simulink model "Qbot_2022a"  (R2023a)
settings: Solver=ode1  StartTime=0.0  StopTime=inf  FixedStep=1/60  RelTol=1e-3
PostLoadFcn:
  | qlabs_setup
model workspace: external: MATLAB File Qbot_2022a_saveas.m (data not in the file)
values from neighbouring files (symbols this model uses):
  D = 0.393    [param.m]
  kd1 = 1    [param.m]
  kd2 = kd1    (= 1)    [param.m]
  kp1 = 2    [param.m]
  kp2 = kp1    (= 2)    [param.m]
  R = 0.04445    [param.m]
  Tinv = inv(T)    [param.m]
  v0 = sqrt(xdr0.^2+ydr0.^2)    [param.m]
  wlmax = wrmax    (= 8)    [param.m]
  wrmax = 8.0    (= 8)    [param.m]
  X0 = [0 0 0]'    [param.m]
libraries: quarc_library x11, dspsigops x1
settings Model: SimulationMode=external  ExtModeTrigDuration=10000  Creator=mbohra  LastModifiedBy=surya
settings DebuggingCC: UnderspecifiedInitializationDetection=Classic  MergeDetectMultiDrivingBlocksExec=none
settings ModelReferenceCC: PropagateSignalLabelsOutOfModel=off

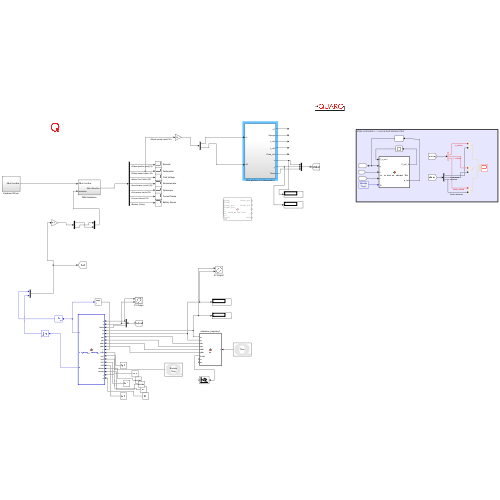
[thumbnail: Simulink's stored preview of the top-level diagram]
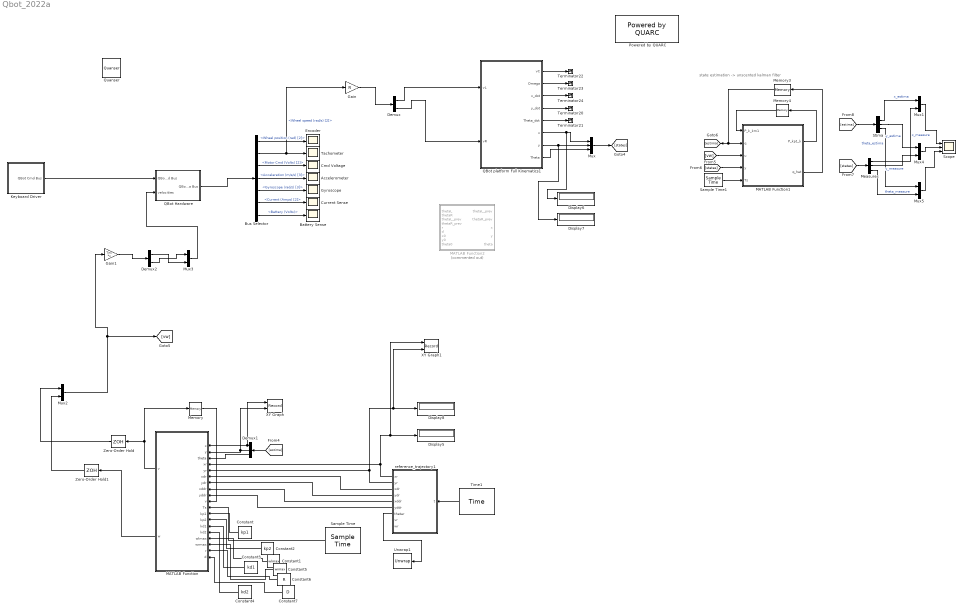
== system Qbot_2022a ==
  note: state estimation -> unscented kalman filter
  Accelerometer : Scope
  Battery Sense : Scope
  Bus Selector : BusSelector  OutputSignals=Wheel position (rad) [2],Wheel speed (rad/s) [2],Motor Cmd (Volts) [2],Acceleration (m/s/s) [3],Gyroscope (rad/s) [3],Current (Amps) [2],Battery (Volts)
  Cmd Voltage : Scope
  Constant : Constant  Value=kp1
  Constant1 : Constant  Value=wlmax
  Constant2 : Constant  Value=kp2
  Constant3 : Constant  Value=kd1
  Constant4 : Constant  Value=kd2
  Constant5 : Constant  Value=wrmax
  Constant6 : Constant  Value=R
  Constant7 : Constant  Value=D
  Current Sense : Scope
  Demux : Demux  Outputs=2
  Demux1 : Demux  Outputs=3
  Demux2 : Demux  Outputs=2
  Display{5..8} (4 alike) : Display
  Encoder : Scope
  Gain : Gain  Gain=R
  Gain1 : Gain  Gain=Tinv  Multiplication=Matrix(K*u)
  Gyroscope : Scope
  Keyboard Driver : Subsystem
  MATLAB Function : MATLAB Function  TreatAsAtomicUnit=on
  MATLAB Function1 : MATLAB Function  TreatAsAtomicUnit=on
  MATLAB Function2 : MATLAB Function  Commented=on  TreatAsAtomicUnit=on
  Measures : Demux  Outputs=3
  Memory : Memory  InitialCondition=v0
  Memory3 : Memory  InitialCondition=X0
  Memory4 : Memory  InitialCondition=1e-3*eye(3)
  Mux : Mux  Inputs=3
  Mux{1..5} (5 alike) : Mux  Inputs=2
  Powered by QUARC : quarc_library/Logos/Powered by QUARC
  QBot Hardware : Subsystem
  QBot platform Full Kinematics1 : Subsystem
  Quanser : quarc_library/Logos/Quanser
  Sample Time : quarc_library/Sources/Time/Sample Time  Priority=-99  sample_time=Ts
  Sample Time1 : quarc_library/Sources/Time/Sample Time  Priority=-99  sample_time=Ts
  Scope : Scope  NumInputPorts=3
  Stima : Demux  Outputs=3
  Tachometer : Scope
  Terminator{20..24} (5 alike) : Terminator
  Time1 : quarc_library/Sources/Time/Time  time_source=Wall clock  sample_time=qc_get_step_size
  Unwrap1 : dspsigops/Unwrap  tol=pi  InputProcessing=Columns as channels (frame based)  running=off
  XY Graph : Record  FileSettingsInternal="{\"entries\":[{\"content\":{\"excelSettings\":{\"content\":{},\"type\":\"Streamout.ExcelSettings\"}},\"type\":\"Streamout.FileSettingStorage\",\"uuid\":\"\"}],\"packageUris\":[\"http:\\/\\/schema.mathworks.com\\/mf0\\/streamout_blocks\\/R2020a\"],\"version\":\"1.0\"}"  Layout=[1 1]  SignalsInternal="{\"entries\":[{\"content\":{\"signals\":[{\"content\":{\"blockPath\":[],\"dimensions\":[1],\"domain\":\"\",\"lineColor\":\"#a2142f\",\"plots\":[1],\"port\":1,\"signalID\":1415,\"signalName\":\"Demux1:1\"},\"type\":\"RecordBlkView.Signal\",\"uuid\":\"\"},{\"content\":{\"blockPath\":[],\"dimensions\":[1],\"domain\":\"\",\"lineColor\":\"#139fff\",\"plots\":[1],\"port\":2,\"signalID\":1418,\"signalName\":\"Demux1:2\"},\"type\":\"RecordBlkView.Signal\",\"uuid\":\"\"}]},\"type\":\"RecordBlkView.InputSignals\",\"uuid\":\"\"}],\"packageUris\":[\"http:\\/\\/schema.mathworks.com\\/mf0\\/streamout_blocks\\/R2020a\"],\"version\":\"1.0\"}"  VisualizationBindings="{\"xyplotplugin\":{\"info\":[{\"series\":[{\"bindingParametersList\":[{\"parameter\":\"X-Axis\",\"signalID\":1415,\"signalName\":\"Demux1:1\"},{\"parameter\":\"Y-Axis\",\"signalID\":1418,\"signalName\":\"Demux1:2\"}],\"seriesID\":17618}],\"subplotID\":1}]}}"  CompatibilityTag=XY
  XY Graph1 : Record  FileSettingsInternal="{\"entries\":[{\"content\":{\"excelSettings\":{\"content\":{},\"type\":\"Streamout.ExcelSettings\"}},\"type\":\"Streamout.FileSettingStorage\",\"uuid\":\"\"}],\"packageUris\":[\"http:\\/\\/schema.mathworks.com\\/mf0\\/streamout_blocks\\/R2020a\"],\"version\":\"1.0\"}"  Layout=[1 1]  SignalsInternal="{\"entries\":[{\"content\":{\"signals\":[{\"content\":{\"blockPath\":[],\"dimensions\":[1],\"domain\":\"\",\"lineColor\":\"#a2142f\",\"plots\":[1],\"port\":1,\"signalID\":1407,\"signalName\":\"reference_trajectory1:1\"},\"type\":\"RecordBlkView.Signal\",\"uuid\":\"\"},{\"content\":{\"blockPath\":[],\"dimensions\":[1],\"domain\":\"\",\"lineColor\":\"#139fff\",\"plots\":[1],\"port\":2,\"signalID\":1410,\"signalName\":\"reference_trajectory1:2\"},\"type\":\"RecordBlkView.Signal\",\"uuid\":\"\"}]},\"type\":\"RecordBlkView.InputSignals\",\"uuid\":\"\"}],\"packageUris\":[\"http:\\/\\/schema.mathworks.com\\/mf0\\/streamout_blocks\\/R2020a\"],\"version\":\"1.0\"}"  VisualizationBindings="{\"xyplotplugin\":{\"info\":[{\"series\":[{\"bindingParametersList\":[{\"parameter\":\"X-Axis\",\"signalID\":1407,\"signalName\":\"reference_trajectory1:1\"},{\"parameter\":\"Y-Axis\",\"signalID\":1410,\"signalName\":\"reference_trajectory1:2\"}],\"seriesID\":30743}],\"subplotID\":1}]}}"  CompatibilityTag=XY
  Zero-Order Hold : ZeroOrderHold  SampleTime=1/60
  Zero-Order Hold1 : ZeroOrderHold  SampleTime=1/60
  reference_trajectory1 : MATLAB Function  TreatAsAtomicUnit=on
  wires:
  Bus Selector/7 -> Battery Sense/1  "<Battery (Volts)>"
  Keyboard Driver/1(QBot Cmd Bus) -> QBot Hardware/1(QBot Cmd Bus)
  Bus Selector/1 -> Encoder/1  "<Wheel position (rad) [2]>"
  Bus Selector/3 -> Cmd Voltage/1  "<Motor Cmd (Volts) [2]>"
  Bus Selector/4 -> Accelerometer/1  "<Acceleration (m/s/s) [3]>"
  QBot Hardware/1(QBot Data Bus) -> Bus Selector/1
  Bus Selector/6 -> Current Sense/1  "<Current (Amps) [2]>"
  Bus Selector/5 -> Gyroscope/1  "<Gyroscope (rad/s) [3]>"
  [estima] -> Demux1/1
  Memory/1 -> MATLAB Function/10("v ")
  reference_trajectory1/5(xddr) -> MATLAB Function/8(xddr)
  Demux1/1 -> XY Graph/1, MATLAB Function/1(x)
  Zero-Order Hold/1 -> Mux2/1
  reference_trajectory1/6(yddr) -> MATLAB Function/9(yddr)
  reference_trajectory1/2(yr) -> XY Graph1/2, Display8/1, MATLAB Function/5(yr)
  Demux1/2 -> XY Graph/2, MATLAB Function/2(y)
  Sample Time/1 -> MATLAB Function/11(Ts)
  reference_trajectory1/4(ydr) -> MATLAB Function/7(ydr)
  Constant4/1 -> MATLAB Function/15(kd2)
  reference_trajectory1/3(xdr) -> MATLAB Function/6(xdr)
  Constant3/1 -> MATLAB Function/14(kd1)
  Constant2/1 -> MATLAB Function/13(kp2)
  Constant/1 -> MATLAB Function/12(kp1)
  reference_trajectory1/1(xr) -> XY Graph1/1, Display5/1, MATLAB Function/4(xr)
  Time1/1 -> reference_trajectory1/1(t)
  MATLAB Function/2(w) -> Zero-Order Hold1/1
  MATLAB Function/1(v) -> Memory/1, Zero-Order Hold/1
  Demux1/3 -> MATLAB Function/3(theta)
  Demux/2 -> QBot platform Full Kinematics1/2(vR)
  QBot platform Full Kinematics1/4(y_dot) -> Terminator20/1
  Demux/1 -> QBot platform Full Kinematics1/1(vL)
  QBot platform Full Kinematics1/6(x) -> Mux/1, Display6/1
  QBot platform Full Kinematics1/8(Theta) -> Mux/3
  Mux/1 -> [states]
  QBot platform Full Kinematics1/2(Omega) -> Terminator23/1
  QBot platform Full Kinematics1/7(y) -> Display7/1, Mux/2
  QBot platform Full Kinematics1/1(vC) -> Terminator22/1
  QBot platform Full Kinematics1/3(x_dot) -> Terminator24/1
  QBot platform Full Kinematics1/5(Theta_dot) -> Terminator21/1
  Gain/1 -> Demux/1
  Bus Selector/2 -> Gain/1, Tachometer/1  "<Wheel speed (rad/s) [2]>"
  MATLAB Function1/1(P_kp1_k) -> Memory4/1
  [states] -> MATLAB Function1/4(y)
  Stima/3 -> Mux5/1  "theta_estima"
  MATLAB Function1/2(q_hat) -> Memory3/1
  Sample Time1/1 -> MATLAB Function1/5(Ts)
  Stima/2 -> Mux4/1  "y_estima"
  Measures/1 -> Mux1/2  "x_measure"
  Measures/2 -> Mux4/2  "y_measure"
  Mux1/1 -> Scope/1
  Memory3/1 -> MATLAB Function1/2(q), [estima]
  Mux5/1 -> Scope/3
  Mux4/1 -> Scope/2
  [states] -> Measures/1
  Measures/3 -> Mux5/2  "theta_measure"
  Stima/1 -> Mux1/1  "x_estima"
  [vw] -> MATLAB Function1/3(u)
  [estima] -> Stima/1
  Memory4/1 -> MATLAB Function1/1(P_k_km1)
  reference_trajectory1/7(thetar) -> Unwrap1/1
  Mux2/1 -> [vw], Gain1/1
  Gain1/1 -> Demux2/1
  Demux2/1 -> Mux3/2
  Demux2/2 -> Mux3/1
  Mux3/1 -> QBot Hardware/2(velocities)
  Zero-Order Hold1/1 -> Mux2/2
  Constant1/1 -> MATLAB Function/16(wlmax)
  Constant5/1 -> MATLAB Function/17(wrmax)
  Constant6/1 -> MATLAB Function/18(r)
  Constant7/1 -> MATLAB Function/19(d)

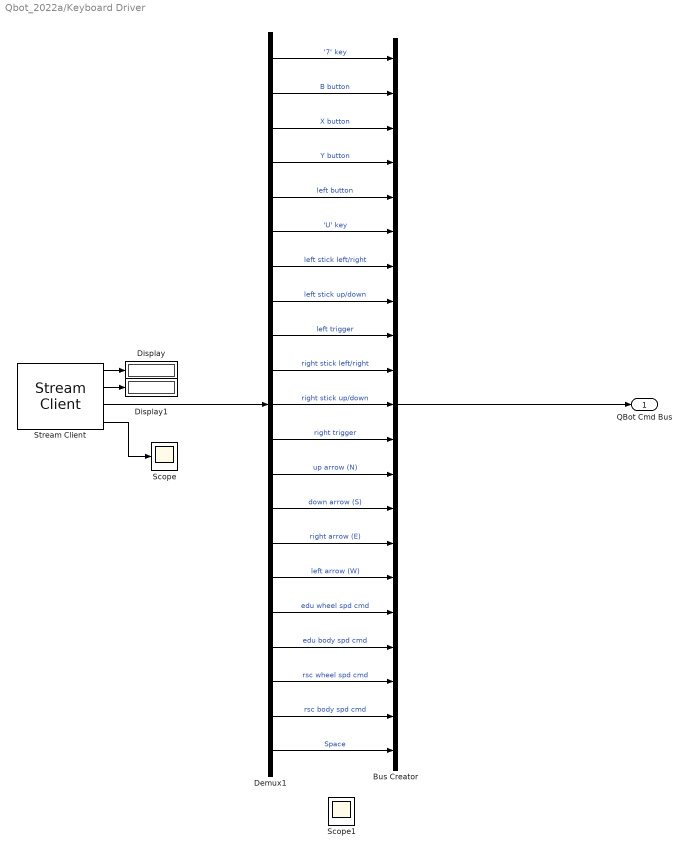
== system Qbot_2022a/Keyboard Driver ==
  Bus Creator : BusCreator  Inputs=21
  Demux1 : Demux  Outputs=[1 1 1 1 1 1 1 1 1 1 1 1 1 1 1 1 2 2 2 2 1]
  Display : Display
  Display1 : Display
  Scope : Scope
  Scope1 : Scope
  Stream Client : quarc_library/Communications/Basic/Stream Client  uri_source=Specify via dialog (do not evaluate)  uri=tcpip://localhost:18889?nagle='off'  send_buffer_size=1460  receive_buffer_size=1460  byte_order=little endian (Intel - LSB first)  optimization=Minimum latency  send_options=Do not send data  receive_options=Receive most recent data  default_value=zeros(25,1)  sample_time=qc_get_step_size  active=on  implementation=Use blocking I/O in a separate thread  send_fifo_size=1000  receive_fifo_size=1000  send_priority=0  receive_priority=0  send_dimensions=off  receive_dimensions=off  max_dimensions=-1  data_type=Inherited via back propagation  type_expr=BusObject
      settings: AttributesFormatString="\"tcpip://localhost:18889?nagle='off'\""
  QBot Cmd Bus : Outport
  wires:
  Bus Creator/1 -> QBot Cmd Bus/1
  Stream Client/3 -> Demux1/1
  Demux1/1 -> Bus Creator/1  "'7' key"
  Demux1/2 -> Bus Creator/2  "B button"
  Demux1/3 -> Bus Creator/3  "X button"
  Demux1/4 -> Bus Creator/4  "Y button"
  Demux1/5 -> Bus Creator/5  "left button"
  Demux1/6 -> Bus Creator/6  "'U' key"
  Demux1/7 -> Bus Creator/7  "left stick left/right"
  Demux1/8 -> Bus Creator/8  "left stick up/down"
  Demux1/9 -> Bus Creator/9  "left trigger"
  Demux1/10 -> Bus Creator/10  "right stick left/right"
  Demux1/11 -> Bus Creator/11  "right stick up/down"
  Demux1/12 -> Bus Creator/12  "right trigger"
  Demux1/13 -> Bus Creator/13  "up arrow (N)"
  Demux1/14 -> Bus Creator/14  "down arrow (S)"
  Demux1/15 -> Bus Creator/15  "right arrow (E)"
  Demux1/16 -> Bus Creator/16  "left arrow (W)"
  Demux1/17 -> Bus Creator/17  "edu wheel spd cmd"
  Demux1/18 -> Bus Creator/18  "edu body spd cmd"
  Demux1/19 -> Bus Creator/19  "rsc wheel spd cmd"
  Demux1/20 -> Bus Creator/20  "rsc body spd cmd"
  Demux1/21 -> Bus Creator/21  "Space"
  Stream Client/1 -> Display/1
  Stream Client/2 -> Display1/1
  Stream Client/4 -> Scope/1

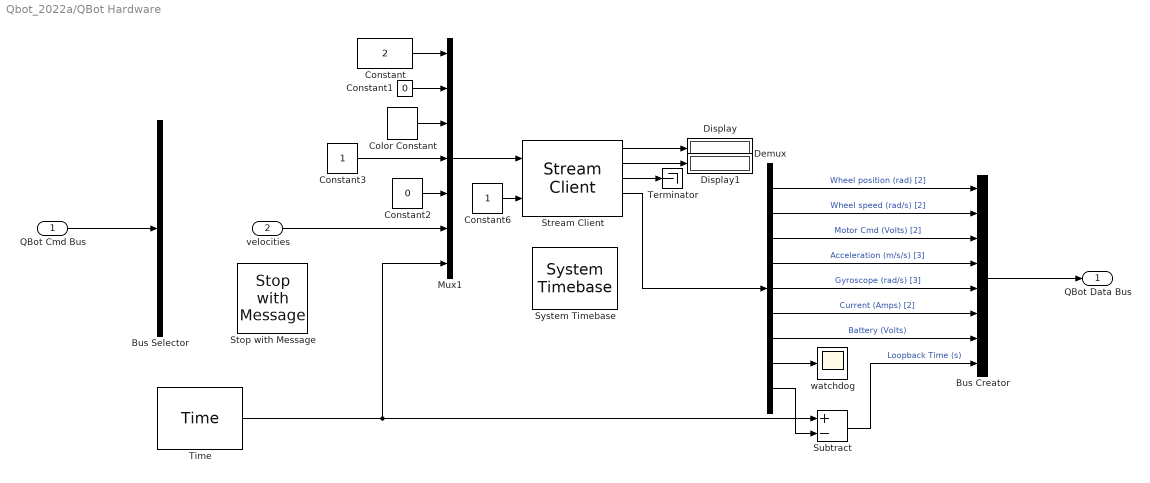
== system Qbot_2022a/QBot Hardware ==
  QBot Cmd Bus : Inport
  velocities : Inport  Port=2
  Bus Creator : BusCreator  Inputs=8
  Bus Selector : BusSelector  OutputSignals=Space,edu body spd cmd,'U' key
  Color Constant : quarc_library/Sources/Signals/Color Constant  color=[0 1 1]
      settings: SourceProductName=QUARC Targets
  Constant : Constant  Value=2
  Constant1 : Constant  Value=0
  Constant2 : Constant  Value=0
  Constant3 : Constant
  Constant6 : Constant
  Demux : Demux  Outputs=[2 2 2 3 3 2 1 1 1]
  Display : Display
  Display1 : Display
  Mux1 : Mux  Inputs=7
  Stop with Message : quarc_library/Sinks/Error Handling/Stop with Message  message_type=Fixed error message  message_icon=Information  message=Operator: Emergency Stop
  Stream Client : quarc_library/Communications/Basic/Stream Client  uri_source=Specify via dialog (do not evaluate)  uri=tcpip://localhost:18888  send_buffer_size=1460  receive_buffer_size=1460  byte_order=little endian (Intel - LSB first)  optimization=Minimum latency  send_options=Send most recent data  receive_options=Receive most recent data  default_value=zeros(17,1)  sample_time=qc_get_step_size  active=on  implementation=Use blocking I/O in a separate thread  send_fifo_size=1000  receive_fifo_size=1000  send_priority=0  receive_priority=0  send_dimensions=off  receive_dimensions=off  max_dimensions=-1  data_type=Inherited via back propagation  type_expr=BusObject
      settings: AttributesFormatString="\"tcpip://localhost:18888\""
  Subtract : Sum  Inputs=+-
  System Timebase : quarc_library/Advanced/Timing/System Timebase  stop_on_overrun=off
      settings: SourceProductName=QUARC Targets
  Terminator : Terminator
  Time : quarc_library/Sources/Time/Time  time_source=Wall clock  sample_time=qc_get_step_size
  watchdog : Scope
  QBot Data Bus : Outport
  wires:
  Demux/2 -> Bus Creator/2  "Wheel speed (rad/s) [2]"
  Constant/1 -> Mux1/1
  Stream Client/3 -> Terminator/1
  Stream Client/1 -> Display/1
  Constant6/1 -> Stream Client/2
  Stream Client/2 -> Display1/1
  Color Constant/1 -> Mux1/3
  Constant1/1 -> Mux1/2
  Demux/3 -> Bus Creator/3  "Motor Cmd (Volts) [2]"
  Mux1/1 -> Stream Client/1
  Stream Client/4 -> Demux/1
  Demux/1 -> Bus Creator/1  "Wheel position (rad) [2]"
  Demux/7 -> Bus Creator/7  "Battery (Volts)"
  Demux/5 -> Bus Creator/5  "Gyroscope (rad/s) [3]"
  Demux/6 -> Bus Creator/6  "Current (Amps) [2]"
  Demux/9 -> Subtract/2
  Constant2/1 -> Mux1/5
  Demux/4 -> Bus Creator/4  "Acceleration (m/s/s) [3]"
  Time/1 -> Subtract/1, Mux1/7
  Bus Creator/1 -> QBot Data Bus/1
  Subtract/1 -> Bus Creator/8  "Loopback Time (s)"
  Demux/8 -> watchdog/1
  QBot Cmd Bus/1 -> Bus Selector/1
  velocities/1 -> Mux1/6
  Constant3/1 -> Mux1/4

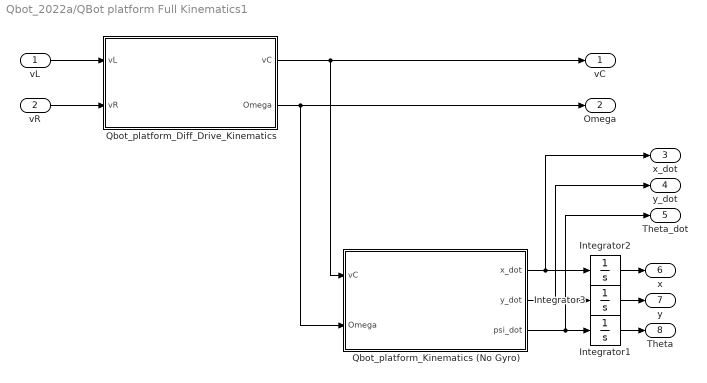
== system Qbot_2022a/QBot platform Full Kinematics1 ==
  vL : Inport
  vR : Inport  Port=2
  Integrator1 : Integrator  InitialCondition=X0(3)
  Integrator2 : Integrator  InitialCondition=X0(1)
  Integrator3 : Integrator  InitialCondition=X0(2)
  Qbot_platform_Diff_Drive_Kinematics : Subsystem
  Qbot_platform_Kinematics (No Gyro) : Subsystem
  vC : Outport  VectorParamsAs1DForOutWhenUnconnected=off
  Omega : Outport  Port=2  VectorParamsAs1DForOutWhenUnconnected=off
  x_dot : Outport  Port=3  VectorParamsAs1DForOutWhenUnconnected=off
  y_dot : Outport  Port=4  VectorParamsAs1DForOutWhenUnconnected=off
  Theta_dot : Outport  Port=5  VectorParamsAs1DForOutWhenUnconnected=off
  x : Outport  Port=6  VectorParamsAs1DForOutWhenUnconnected=off
  y : Outport  Port=7  VectorParamsAs1DForOutWhenUnconnected=off
  Theta : Outport  Port=8  VectorParamsAs1DForOutWhenUnconnected=off
  wires:
  Integrator1/1 -> Theta/1
  Qbot_platform_Kinematics (No Gyro)/3(psi_dot) -> Theta_dot/1, Integrator1/1
  Qbot_platform_Kinematics (No Gyro)/1(x_dot) -> x_dot/1, Integrator2/1
  Qbot_platform_Kinematics (No Gyro)/2(y_dot) -> y_dot/1, Integrator3/1
  Qbot_platform_Diff_Drive_Kinematics/1(vC) -> Qbot_platform_Kinematics (No Gyro)/1(vC), vC/1
  vL/1 -> Qbot_platform_Diff_Drive_Kinematics/1(vL)
  vR/1 -> Qbot_platform_Diff_Drive_Kinematics/2(vR)
  Integrator2/1 -> x/1
  Integrator3/1 -> y/1
  Qbot_platform_Diff_Drive_Kinematics/2(Omega) -> Qbot_platform_Kinematics (No Gyro)/2(Omega), Omega/1

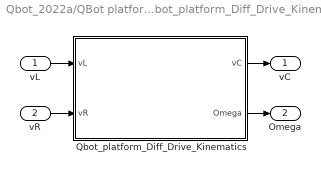
== system Qbot_2022a/QBot platform Full Kinematics1/Qbot_platform_Diff_Drive_Kinematics ==
  vL : Inport
  vR : Inport  Port=2
  Qbot_platform_Diff_Drive_Kinematics : MATLAB Function  TreatAsAtomicUnit=on
  vC : Outport  VectorParamsAs1DForOutWhenUnconnected=off
  Omega : Outport  Port=2  VectorParamsAs1DForOutWhenUnconnected=off
  wires:
  vL/1 -> Qbot_platform_Diff_Drive_Kinematics/1(vL)
  Qbot_platform_Diff_Drive_Kinematics/1(vC) -> vC/1
  vR/1 -> Qbot_platform_Diff_Drive_Kinematics/2(vR)
  Qbot_platform_Diff_Drive_Kinematics/2(Omega) -> Omega/1

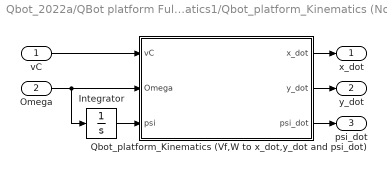
== system Qbot_2022a/QBot platform Full Kinematics1/Qbot_platform_Kinematics (No Gyro) ==
  vC : Inport
  Omega : Inport  Port=2
  Integrator : Integrator
  Qbot_platform_Kinematics (Vf,W to x_dot,y_dot and psi_dot) : MATLAB Function  TreatAsAtomicUnit=on
  x_dot : Outport  VectorParamsAs1DForOutWhenUnconnected=off
  y_dot : Outport  Port=2  VectorParamsAs1DForOutWhenUnconnected=off
  psi_dot : Outport  Port=3  VectorParamsAs1DForOutWhenUnconnected=off
  wires:
  Qbot_platform_Kinematics (Vf,W to x_dot,y_dot and psi_dot)/3(psi_dot) -> psi_dot/1
  Integrator/1 -> Qbot_platform_Kinematics (Vf,W to x_dot,y_dot and psi_dot)/3(psi)
  vC/1 -> Qbot_platform_Kinematics (Vf,W to x_dot,y_dot and psi_dot)/1(vC)
  Qbot_platform_Kinematics (Vf,W to x_dot,y_dot and psi_dot)/1(x_dot) -> x_dot/1
  Omega/1 -> Integrator/1, Qbot_platform_Kinematics (Vf,W to x_dot,y_dot and psi_dot)/2(Omega)
  Qbot_platform_Kinematics (Vf,W to x_dot,y_dot and psi_dot)/2(y_dot) -> y_dot/1

== matlab function Qbot_2022a/MATLAB Function2 ==
  data: thetaL_prev output; thetaR_prev output; x output; thetaL input; y output; thetaR input; thetaL_prev input; thetaR_prev input; r input; d input; x0 input; y0 input; theta0 input; theta output
function [thetaL_prev, thetaR_prev,x,y,theta]=computeOdometry(thetaL,thetaR,thetaL_prev, thetaR_prev,r,d,x0,y0,theta0)
    delta_sL=r*(thetaL - thetaL_prev);
    delta_sR=r*(thetaR - thetaR_prev);
    delta_theta=(delta_sR-delta_sL)/d;
    delta_s=(delta_sR+delta_sL)/2;
    theta=theta0+delta_theta/2;
    x=x0+delta_s*cos(theta);
    y=y0+delta_s*sin(theta); 
    thetaL_prev = thetaL;
    thetaR_prev = thetaR;
end

== matlab function Qbot_2022a/reference_trajectory1 ==
  data: xr output; yr output; t input; xdr output; ydr output; xddr output; yddr output; thetar output; vr output; wr output
function [xr, yr,xdr,ydr,xddr,yddr,thetar,vr,wr] = fcn(t)
    eta=1;
    alpha=4;
    % Calculate the current trajectory point
    xr = eta * sin(t / alpha);           % Calculate xr at current time
    yr = eta * sin(t / (2 * alpha));     % Calculate yr at current time
    
    
    
    %Velocity trajectory
    xdr=eta*cos(t / alpha)*(1/alpha); %trajectory velocity along x axis
    ydr=eta*cos(t / (2 * alpha))*(1/(2*alpha));%trajectory velocity along y axis
    
    %Acceleration trajectory
    xddr=-eta*sin(t / alpha)*(1/alpha)*(1/alpha); %trajetcory acceleration along x axis
    yddr=-eta*sin(t / (2 * alpha))*(1/(2*alpha))*(1/(2*alpha));%trajetcory acceleration y axis
    
    % Orientation reference
    thetar=atan2(ydr,xdr); %Trajectory Orientation
    
    vr=sqrt(xdr^2+ydr^2); %Linear velocity of the trajectory
    wr=(yddr*xdr-xddr*ydr)/(xdr^2+ydr^2); %Angular velocity velocity of the trajectory
end

== matlab function Qbot_2022a/MATLAB Function1 ==
  data: P_k_km1 input; P_kp1_k output; q input; u input; q_hat output; y input; Ts input
function [P_kp1_k,q_hat]= my_unscented_kalman_filter(P_k_km1,q,u,y,Ts)
Q=1e-5*eye(3);
R=1e-4*eye(3);
alpha=0.9; beta=2; kappa=0;
%Calculate the Sigma points
M=3;
c=alpha^2*(M+kappa);
q_hat_i=zeros(M,2*M+1);
q_hat_i(:,1)=q;
Delta_x=real(sqrtm(c*P_k_km1));
for i=1:M
    q_hat_i(:,i+1)=q+Delta_x(:,i);
    q_hat_i(:,i+1+M)=q-Delta_x(:,i);
end
%Output of the sigma points
y_hat_i=q_hat_i(1:3,:);
%predicted measurement at time k
W_M=zeros(1,2*M+1);
W_M(1)=1-(M/(alpha^2*(M+kappa)));
W_M(2:2*M+1)=(1/(2*alpha^2*(M+kappa)));
y_k=zeros(3,1);
for i=1:2*M+1
    y_k=y_k+W_M(i)*y_hat_i(:,i);
end
%Estimate of the covariance of predicted measurement
W_c=zeros(1,2*M+1);
W_c(1)=(2-alpha^2+beta)-(M/(alpha^2*(M+kappa)));
W_c(2:2*M+1)=(1/(2*alpha^2*(M+kappa)));
P_y=zeros(3,3);
for i=1:2*M+1
    P_y=P_y+W_c(i)*(y_hat_i(:,i)-y_k)*(y_hat_i(:,i)-y_k)'+R;
end
%%Estimate of the cross-covariance between predicted x and y
P_xy=zeros(M,3);
for i=1:2*M+1
    P_xy=P_xy+(1/(2*alpha^2*(M+kappa)))*(q_hat_i(:,i)-q)*(y_hat_i(:,i)-y_k)';
end
%Kalman gain
K=P_xy/(P_y);
q_k_k = q+K*(y-y_k);
P_k_k = P_k_km1 -K*P_y*K';
% State prediction and state estimation error covariance
q_hat_i_k_k=zeros(M,2*M+1);
q_hat_i_k_k(:,1)=q_k_k;
Delta_x=real(sqrtm(c*P_k_k));
for i=1:M
    q_hat_i_k_k(:,i+1)=q_k_k+Delta_x(:,i);
    q_hat_i_k_k(:,i+1+M)=q_k_k-Delta_x(:,i);
end
%Predicted state for each sigma point
q_hat_kp1_k=zeros(M,2*M+1);
for i=1:2*M+1
    q_hat_kp1_k(:,i)=q_hat_i_k_k(:,i)+Ts*[cos(q_hat_i_k_k(3,i)) 0;
        sin(q_hat_i_k_k(3,i)) 0;
        0          1]*u;
end
%Predicted state k+1 at time k
q_hat=zeros(M,1);
for i=1:2*M+1
    q_hat=q_hat + W_M(i)*q_hat_kp1_k(:,i);
end
%Covariance of the predicted state
P_kp1_k=zeros(M,M);
for i=1:2*M+1
    P_kp1_k=P_kp1_k+W_c(i)*(q_hat_kp1_k(:,i)-q_hat)*(q_hat_kp1_k(:,i)-q_hat)'+Q;
end
end

== matlab function Qbot_2022a/QBot platform Full Kinematics1/Qbot_platform_Diff_Drive_Kinematics/Qbot_platform_Diff_Drive_Kinematics ==
  data: vL input; vC output; vR input; Omega output
function [vC,Omega] = fcn(vL,vR)
%#codegen

d= 0.393;

vC=0.5*(vL+vR);
Omega=(1/d)*(vR-vL);

== matlab function Qbot_2022a/QBot platform Full Kinematics1/Qbot_platform_Kinematics (No Gyro)/Qbot_platform_Kinematics (Vf,W to x_dot,y_dot and psi_dot) ==
  data: vC input; x_dot output; Omega input; y_dot output; psi input; psi_dot output
function [x_dot,y_dot,psi_dot] = fcn(vC,Omega,psi)
%#codegen


x_dot=cos(psi)*vC;
y_dot=sin(psi)*vC;
psi_dot= Omega;

== matlab function Qbot_2022a/MATLAB Function ==
  data: x input; v output; y input; theta input; xr input; yr input; w output; xdr input; ydr input; xddr input; yddr input; v input; Ts input; kp1 input; kp2 input; kd1 input; kd2 input; wlmax input; wrmax input; r input; d input
function [v,w] = Trajectory_Tracking_law(x,y,theta,xr,yr,xdr,ydr,xddr,yddr,v,Ts,kp1,kp2,kd1,kd2, wlmax,wrmax,r,d)

    %This function implements the feedback linearization based tracking
    %controller proposed in: "De Luca, Oriolo, Vendittelli - Control of Wheeled Mobile Robots: An
    %Experimental Overview" Section 5.4 - formula 5.18
    
    %xr,yr,xdr,ydr,xddr,yddr, are the positions, velocities, and
    %accelerations of the reference trajectory along the x and y axis
    
    %x,y,theta is the state of the differential-drive/unicycle robot
     
    %Ts is the sampling time
    
    %kp1,kp2,kd1,kd2 are designing parameters
    
    %the outputs v and w are the control linear and angular velocities of
    %unicyle robot

    xd=v*cos(theta);
    yd=v*sin(theta);
    
    u1=xddr+kp1*(xr-x)+kd1*(xdr-xd);
    u2=yddr+kp2*(yr-y)+kd2*(ydr-yd);
    
    a=u1*cos(theta)+u2*sin(theta);
    
    
    v=v+a*Ts;
    
    
    w=(u2*cos(theta)-u1*sin(theta))/v;
    [v,w]=unicycle_saturation(wrmax,wlmax,v,w,r,d);
    

end


function [v,w] = unicycle_saturation(wrmax,wlmax,v,w,r,d)
    
    if w>2*wrmax*r/d
        w=2*wrmax*r/d;
    end
    if w<-(2*wrmax*r/d)
        w=-2*wrmax*r/d;
    end
    
    if v>r*wrmax-d/2*w
        v=r*wrmax-d/2*w;
    end
    if v>r*wlmax+d/2*w
        v=r*wlmax+d/2*w;
    end
    
    if v<-(r*wrmax-d/2*w)
        v=-(r*wrmax-d/2*w);
    end
    if v<-(r*wlmax+d/2*w)
        v=-(r*wlmax+d/2*w);
    end
end
